simulink model "Drone_Simulation"  (R2020a)
settings: Solver=ode1  StartTime=0.0  StopTime=15  FixedStep=1e-3
undefined symbols (not defined in the file): AeEMSC, alpha1TDDBSC, B, bBNG, bEMSC, bEVCAP, BNG_Motor1, BNG_Motor2, BNG_Motor3, BNG_Motor4, BNG_Motor5, BNG_Motor6, bp, bq, br, bTDDBSC, bWDG, C_A, C_mot, C_th_esc, CAPEV_Motor1, CAPEV_Motor2, CAPEV_Motor3, CAPEV_Motor4, CAPEV_Motor5, CAPEV_Motor6, cdx, cdy, cdz, EaEMSC, EaEVCAP, EalphaTDDBSC, EaTDDBSC, EaWDG, FuselageContactForces, g, JrefEMSC, k_b, Kp, Kp2, Kq, Kq2, Kr, Kr2, kv, Kx, Ky, Kz, Kz2, LeftAftArm, LeftAftSkid, LeftArm, LeftFrontArm, LeftFrontSkid, LeftSideContactForces, LnomEMSC, LnomEVCAP, LnomTDDBSC, LnomWDG, Lower ... (+65)
libraries: sm_lib x90, nesl_utility x76, fl_lib x59, ee_lib x18, batteryecm_lib x2, dspinverses x1, dspmtrx3 x1
(part 1 of 5)
settings Model: Creator=G_MAMAN  LastModifiedBy=Asus
settings SolverCC: MaxConsecutiveZCs=100  ExtrapolationOrder=2  AlgebraicLoopSolver=LineSearch  SolverResetMethod=Robust
settings DataIOCC: LimitDataPoints=on  MaxDataPoints=10000  Refine=5
settings OptimizationCC: LifeSpan=inf
settings DebuggingCC: MaskedZcDiagnostic=none  IgnoredZcDiagnostic=none  AllowSymbolicDim=off  SFUnexpectedBacktrackingDiag=warning  SFNoUnconditionalDefaultTransitionDiag=warning  SFExecutionAtInitializationDiag=none  ArithmeticOperatorsInVariantConditions=warning
settings SFSimCC: SimUseLocalCustomCode=off  CustomCodeUndefinedFunction=UseInterfaceOnly
settings RTWCC: RTWUseLocalCustomCode=off
settings CodeAppCC: StateflowObjectComments=on
settings GRTTargetCC: TargetLangStandard=C89/C90 (ANSI)
settings ConfigComp: CovMetricSettings=dw  CovSaveCumulativeToWorkspaceVar=on  CovSaveSingleToWorkspaceVar=on  CovExternalEMLEnable=off  CovSFcnEnable=off
settings SimscapeCC: ExplicitSolverDiagnosticOptions=none  SimscapeLogType=all  SimscapeLogSimulationStatistics=on  SimscapeLogDataHistory=10000
settings DiagnosticsConfigSet: SimMechanicsRigidlyBoundBlock=none
settings ExplorerConfigSet: InternalSimMechanicsExplorerSettings="<ExplorerConfiguration><canonicalview>default</canonicalview><AnimationSetting><BasePlaybackSpeed>1.0</BasePlaybackSpeed><PlaybackSpeedFactor>1.0</PlaybackSpeedFactor></AnimationSetting><TilePanel><TileInfo><Tiles Columns=\"1\" Count=\"1\" Rows=\"1\"><Column Weight=\"1\"/><Row Weight=\"1\"/><Tile Height=\"1\" Width=\"1\" X=\"0\" Y=\"0\"/></Tiles></TileInfo><SceneInfo><SceneViewer><BGColor><R>0</R><G>0</G><B>0</B></BGColor><Camera><DoPerspective>off</DoPerspective><Position><X>7.1395388580893373</X><Y>-9.57545541238177833</Y><Z>5.80767107239631564</Z></Position><Center><X>-0.863567299281931766</X><Y>0.176174380151177173</Y><Z>1.92916926391305155</Z></Center><Up><X>-0.173509302469238902</X><Y>0.237715937307242831</Y><Z>0.955712119367949198</Z></Up><ViewLimDist>1</ViewLimDist><YLim>4.19925208742349287</YLim><XLim>9.96419089960335391</XLim></Camera></SceneViewer></SceneInfo></TilePanel><MechEditorPanel><Cameras/><GfxPanelCameraMap/><VideoCreator><PlaybackSpeedRatio>1.0</PlaybackSpeedRatio><FrameRate>30</FrameRate><VideoFormat>Motion JPEG AVI</VideoFormat><FrameSize>auto</FrameSize></VideoCreator></MechEditorPanel></ExplorerConfiguration>"

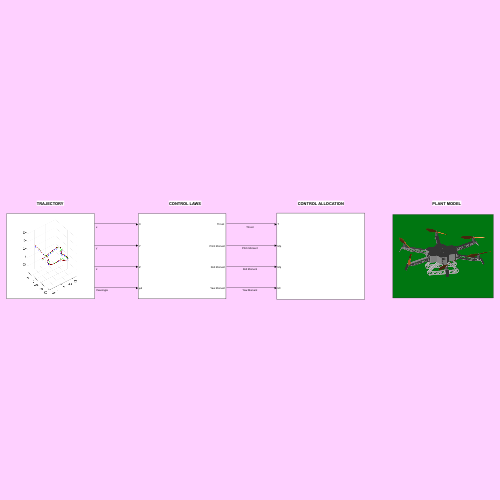
[thumbnail: Simulink's stored preview of the top-level diagram]
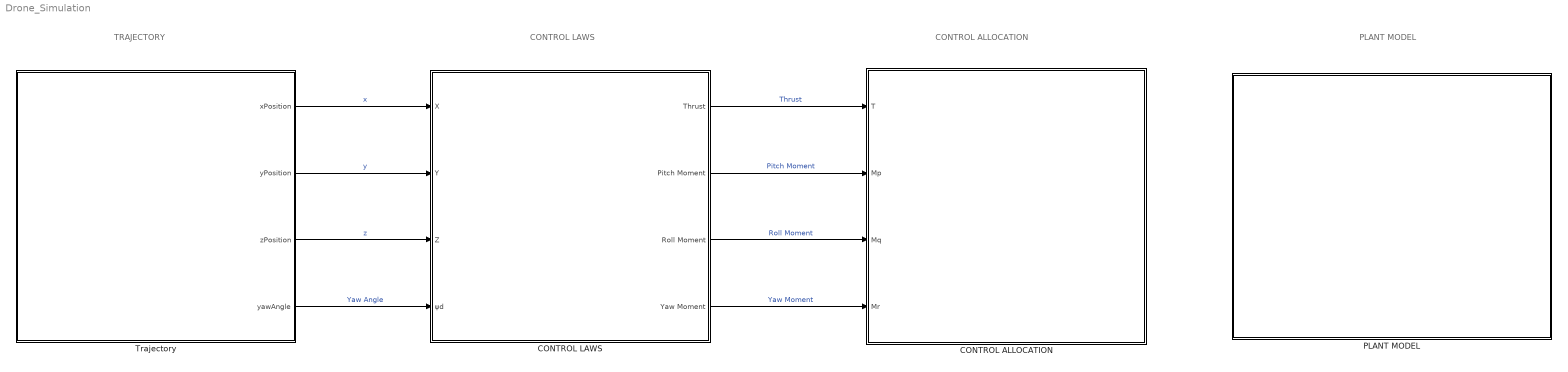
== system Drone_Simulation ==
  note: CONTROL LAWS
  note: CONTROL ALLOCATION
  note: PLANT MODEL
  note: TRAJECTORY
  CONTROL ALLOCATION : Subsystem
  CONTROL LAWS : Subsystem
  PLANT MODEL : Subsystem
      mask Display: image('$imagefile'); % Use "Edit Image" on toolstrip to change.
  Trajectory : Subsystem
      mask Display: image('$imagefile'); % Use "Edit Image" on toolstrip to change.
  wires:
  CONTROL LAWS/4(Yaw Moment) -> CONTROL ALLOCATION/4(Mr)  "Yaw Moment"
  CONTROL LAWS/2(Pitch Moment) -> CONTROL ALLOCATION/2(Mp)  "Pitch Moment"
  CONTROL LAWS/1("Thrust ") -> CONTROL ALLOCATION/1(T)  "Thrust"
  CONTROL LAWS/3(Roll Moment) -> CONTROL ALLOCATION/3(Mq)  "Roll Moment"
  Trajectory/1(xPosition) -> CONTROL LAWS/1(X)  "x"
  Trajectory/2(yPosition) -> CONTROL LAWS/2(Y)  "y"
  Trajectory/3(zPosition) -> CONTROL LAWS/3(Z)  "z"
  Trajectory/4(yawAngle) -> CONTROL LAWS/4(ψd)  "Yaw Angle"

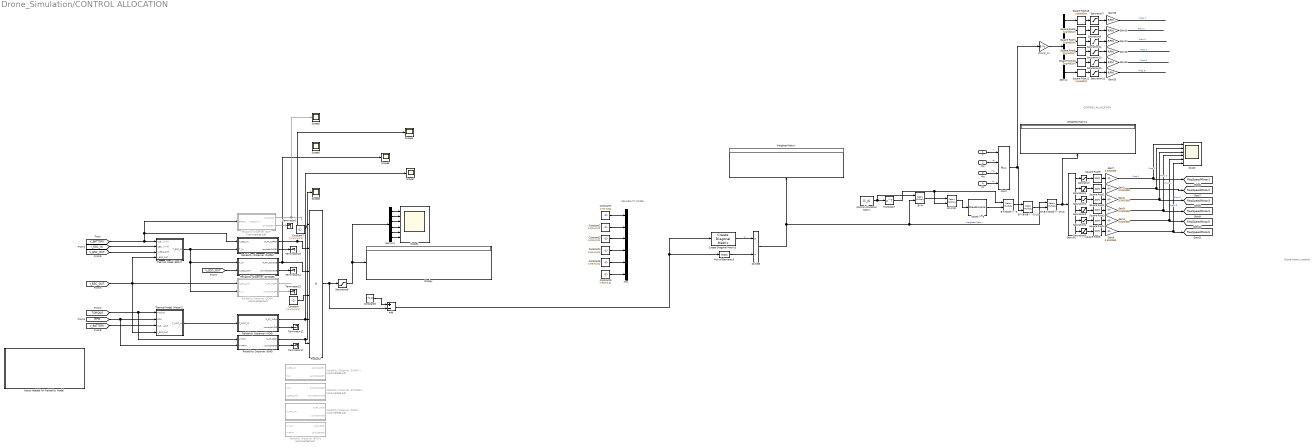
== system Drone_Simulation/CONTROL ALLOCATION ==
  note: Drone Motors Location
  note: RELIABILITY MODEL
  note: CONTROL ALLOCATION
  T : Inport
  Mp : Inport  Port=2
  Mq : Inport  Port=3
  Mr : Inport  Port=4
  (BWB')^-3 : dspinverses/Pseudoinverse  wanterr=off  SimulateUsing=Interpreted execution
  Add : Sum  Inputs=+-
  B'*(BWB')^-1*U3 : Product  Multiplication=Matrix(*)
  B'*(BWB')^-3 : Product  Multiplication=Matrix(*)
  B*W : Product  Multiplication=Matrix(*)
  B*W*B' : Product  Multiplication=Matrix(*)
  Constant : Constant  Value=[1,1,1,1,1,1]
  Constant1 : Constant  Value=1-R1+eps
  Constant2 : Constant  Value=1-R2+0.01
  Constant3 : Constant  Value=1-R3+0.01
  Constant4 : Constant  Value=1-R4+0.01
  Constant5 : Constant  Value=1-R5+0.01
  Constant6 : Constant  Value=1-R6+0.01
  Constant7 : Constant  Value=[1,1,1,1,1,1]
  Constant8 : Constant  Value=1+0.01
  Control Allocation Matrix : Constant  Value=[C_A]
  Create Diagonal Matrix3 : dspmtrx3/Create Diagonal Matrix
  Demux : Demux  Outputs=6
  Demux1 : Demux  Outputs=6
  Demux2 : Demux  Outputs=6
  Display : Display
  Divide3 : Product  Inputs=*/
  Gain{1..5,7} (6 alike) : Gain  Gain=9.5492968
  Gain{15..20} (6 alike) : Gain  Gain=RPM
  Inputs Needed For Reliability Model : Subsystem
  Max of Elements3 : MinMax  Function=max
  Mux : Mux  Inputs=6
  Mux2 : Mux
      settings: DisplayOption=signals
  Pinv(C_A) : Gain  Gain=B  Multiplication=Matrix(K*u)
  Product2 : Product  Inputs=6
  Reliability Observer (BAT) : Subsystem  Commented=on
  Reliability Observer (BNG) : Subsystem
  Reliability Observer (BNG)1 : Subsystem  Commented=on
  Reliability Observer (CAPEV) : Subsystem
  Reliability Observer (CAPEV)1 : Subsystem  Commented=on
  Reliability Observer (SCEM) : Subsystem  Commented=on
  Reliability Observer (SCTDDB) : Subsystem
  Reliability Observer (SCTDDB)1 : Subsystem  Commented=on
  Reliability Observer (WDG) : Subsystem
  Reliability Observer (WDG)1 : Subsystem  Commented=on
  Saturation{,1..5} (6 alike) : Saturate  UpperLimit=1096623  LowerLimit=0
  Saturation{7,9..13} (6 alike) : Saturate  UpperLimit=10000*(2*pi)/60  LowerLimit=0
  Saturation8 : Saturate  UpperLimit=1  LowerLimit=0.01
  Scope : Scope  NumInputPorts=6
  Scope1 : Scope  NumInputPorts=6
  Scope{3..8} (6 alike) : Scope
  Square Root{1..5,9} (6 alike) : Sqrt  SaturateOnIntegerOverflow=on
  Square Root{6..8,10..11,18} (6 alike) : Sqrt  Operator=signedSqrt  SaturateOnIntegerOverflow=on
  Terminator{1,12..15,17} (6 alike) : Terminator
  Thermal Model (ESC)2 : Subsystem
  Thermal Model (Motor)2 : Subsystem
  Transpose : Math  Operator=transpose  SaturateOnIntegerOverflow=on
  W*B'*(BWB')^-1*U3 : Product  Multiplication=Matrix(*)
  Weighted Matrix : Display
  Weighted Matrix1 : Display
  tag scope: ReqSpeedMotor1=global, ReqSpeedMotor2=global, ReqSpeedMotor3=global, ReqSpeedMotor4=global, ReqSpeedMotor5=global, ReqSpeedMotor6=global
  wires:
  B'*(BWB')^-1*U3/1 -> W*B'*(BWB')^-1*U3/2
  [RPM] -> Reliability Observer (BNG)/2(N (RPM)), Thermal Model (Motor)2/2(RPM)
  Thermal Model (Motor)2/1(T_MOT_IN) -> Reliability Observer (WDG)/1(T_MOT_IN)
  Demux2/6 -> Saturation5/1
  [V_BATTERY] -> Reliability Observer (CAPEV)/1(V_ESC_IN), Reliability Observer (BAT)/1(Battery Voltage (V)), Thermal Model (ESC)2/1(V_ESC_in (V))
  [I_ESC_IN] -> Thermal Model (ESC)2/2(I_ESC_in (A))
  [I_ESC_OUT] -> Reliability Observer (SCEM)/1(I_ESC_OUT), Thermal Model (ESC)2/4(I_ESC_OUT), Thermal Model (Motor)2/4(I_ESC_OUT)
  Square Root4/1 -> Gain4/1
  Demux2/2 -> Saturation1/1
  Mux2/1 -> Pinv(C_A)/1, B'*(BWB')^-1*U3/2
  [V_BATTERY] -> Thermal Model (Motor)2/3(V_ESC_OUT)
  Reliability Observer (SCEM)/2(LambdaSCEM) -> Terminator13/1
  Create Diagonal Matrix3/1 -> Divide3/1  "W"
  Square Root5/1 -> Gain5/1
  Transpose/1 -> B*W*B'/2, B'*(BWB')^-3/1
  B'*(BWB')^-3/1 -> B'*(BWB')^-1*U3/1
  Square Root3/1 -> Gain3/1
  [V_ESC_OUT] -> Thermal Model (ESC)2/3(V_ESC_OUT)
  Gain7/1 -> [ReqSpeedMotor1], Scope/1  "Prop 1"
  Reliability Observer (WDG)/2(LambdaWDG) -> Terminator12/1
  Demux2/4 -> Saturation3/1
  Reliability Observer (BNG)/2(LambdaBNG) -> Terminator17/1
  Control Allocation Matrix/1 -> B*W/1, Transpose/1
  Demux2/1 -> Saturation/1
  Reliability Observer (CAPEV)/2(LambdaCAPEV) -> Terminator15/1
  Gain3/1 -> [ReqSpeedMotor4], Scope/4  "Prop 4"
  Gain5/1 -> [ReqSpeedMotor6], Scope/6  "Prop 6"
  Gain4/1 -> [ReqSpeedMotor5], Scope/5  "Prop 5"
  [TORQUE] -> Reliability Observer (BNG)/1(M (Nm)), Thermal Model (Motor)2/1(Torque)
  Square Root1/1 -> Gain1/1
  Gain2/1 -> [ReqSpeedMotor3], Scope/3  "Prop 3"
  (BWB')^-3/1 -> B'*(BWB')^-3/2
  B*W/1 -> B*W*B'/1
  Square Root2/1 -> Gain2/1
  Gain1/1 -> [ReqSpeedMotor2], Scope/2  "Prop 2"
  Demux2/5 -> Saturation4/1
  Square Root9/1 -> Gain7/1
  Thermal Model (ESC)2/1(T_ESC_IN) -> Reliability Observer (CAPEV)/2(T_IN), Reliability Observer (SCTDDB)/1(T_IN), Reliability Observer (SCEM)/2(T_IN)
  Demux2/3 -> Saturation2/1
  Max of Elements3/1 -> Divide3/2
  Reliability Observer (SCTDDB)/2(LambdaSCTDDB) -> Terminator14/1
  Divide3/1 -> Weighted Matrix/1, B*W/2, W*B'*(BWB')^-1*U3/1  "Weighted Matrix"
  B*W*B'/1 -> (BWB')^-3/1
  Saturation/1 -> Square Root9/1
  Saturation1/1 -> Square Root1/1
  Saturation2/1 -> Square Root2/1
  Saturation3/1 -> Square Root3/1
  Saturation4/1 -> Square Root4/1
  Saturation5/1 -> Square Root5/1
  W*B'*(BWB')^-1*U3/1 -> Weighted Matrix1/1, Demux2/1
  T/1 -> Mux2/1  "T"
  Mp/1 -> Mux2/2  "Mp"
  Mq/1 -> Mux2/3  "Mq"
  Mr/1 -> Mux2/4  "Mr"
  [V_ESC_OUT] -> Reliability Observer (SCTDDB)/2(V_ESC_OUT)
  Reliability Observer (CAPEV)/1(R_RT_CAPEV) -> Scope4/1, Product2/2
  Reliability Observer (SCTDDB)/1(R_RT_SCTDDB) -> Product2/3, Scope6/1
  Reliability Observer (BNG)/1(R_RT_BNG) -> Scope8/1, Product2/6
  Reliability Observer (WDG)/1(R_RT_WDG) -> Scope7/1, Product2/5
  Reliability Observer (BAT)/2(LambdaBAT) -> Terminator1/1
  Reliability Observer (BAT)/1(R_RT_BAT) -> Scope3/1
  Constant/1 -> Product2/4
  Product2/1 -> Add/2, Saturation8/1
  Saturation11/1 -> Gain20/1
  Saturation10/1 -> Gain19/1
  Saturation9/1 -> Gain16/1
  Saturation13/1 -> Gain18/1
  Saturation12/1 -> Gain17/1
  Square Root6/1 -> Saturation9/1
  Square Root18/1 -> Saturation7/1
  Square Root8/1 -> Saturation13/1
  Square Root10/1 -> Saturation10/1
  Saturation7/1 -> Gain15/1
  Demux/4 -> Square Root8/1
  Demux/6 -> Square Root11/1
  Square Root11/1 -> Saturation11/1
  Demux/3 -> Square Root7/1
  Square Root7/1 -> Saturation12/1
  Demux/5 -> Square Root10/1
  Pinv(C_A)/1 -> Demux/1
  Demux/1 -> Square Root18/1
  Demux/2 -> Square Root6/1
  Gain15/1 -> ?  "Prop 1"
  Gain16/1 -> ?  "Prop 2"
  Gain17/1 -> ?  "Prop 3"
  Gain18/1 -> ?  "Prop 4"
  Gain19/1 -> ?  "Prop 5"
  Gain20/1 -> ?  "Prop 6"
  Constant4/1 -> Mux/4
  Constant2/1 -> Mux/2
  Constant1/1 -> Mux/1
  Constant3/1 -> Mux/3
  Constant6/1 -> Mux/6
  Constant5/1 -> Mux/5
  Saturation8/1 -> Demux1/1, Display/1
  Reliability Observer (SCEM)/1(R_RT_SCEM) -> ?
  Demux1/1 -> Scope1/1
  Demux1/2 -> Scope1/2
  Demux1/3 -> Scope1/3
  Demux1/4 -> Scope1/4
  Demux1/5 -> Scope1/5
  Demux1/6 -> Scope1/6
  Constant7/1 -> Product2/1
  Constant8/1 -> Add/1
  Add/1 -> Max of Elements3/1, Create Diagonal Matrix3/1

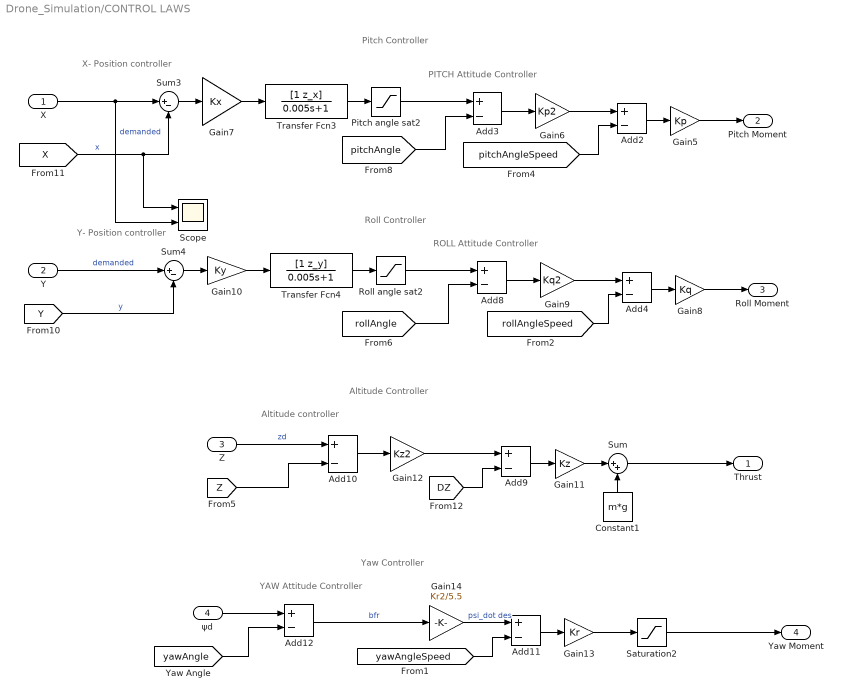
== system Drone_Simulation/CONTROL LAWS ==
  note: PITCH Attitude Controller
  note: X- Position controller
  note: YAW Attitude Controller
  note: Y- Position controller
  note: ROLL Attitude Controller
  note: Altitude controller
  note: Pitch Controller
  note: Roll Controller
  note: Altitude Controller
  note: Yaw Controller
  X : Inport
  Y : Inport  Port=2
  Z : Inport  Port=3
  ψd : Inport  Port=4
  Add{2..4,8..12} (8 alike) : Sum  Inputs=+-
  Constant1 : Constant  Value=m*g
  Gain10 : Gain  Gain=Ky
  Gain11 : Gain  Gain=Kz
  Gain12 : Gain  Gain=Kz2
  Gain13 : Gain  Gain=Kr
  Gain14 : Gain  Gain=Kr2/5.5
  Gain5 : Gain  Gain=Kp
  Gain6 : Gain  Gain=Kp2
  Gain7 : Gain  Gain=Kx
  Gain8 : Gain  Gain=Kq
  Gain9 : Gain  Gain=Kq2
  Pitch angle sat2 : Saturate  UpperLimit=pitch_angle_limit  LowerLimit=-pitch_angle_limit
  Roll angle sat2 : Saturate  UpperLimit=roll_angle_limit  LowerLimit=-roll_angle_limit
  Saturation2 : Saturate  UpperLimit=max_yaw_moment  LowerLimit=-max_yaw_moment
  Scope : Scope  NumInputPorts=2
  Sum : Sum  Inputs=|++
  Sum3 : Sum  Inputs=|+-
  Sum4 : Sum  Inputs=|+-
  Transfer Fcn3 : TransferFcn  Numerator=[1 z_x]  Denominator=[0.005 1]
  Transfer Fcn4 : TransferFcn  Numerator=[1 z_y]  Denominator=[0.005 1]
  "Thrust " : Outport
  Pitch Moment : Outport  Port=2
  Roll Moment : Outport  Port=3
  Yaw Moment : Outport  Port=4
  wires:
  Sum4/1 -> Gain10/1
  Add10/1 -> Gain12/1
  Add9/1 -> Gain11/1
  Add11/1 -> Gain13/1
  [DZ] -> Add9/2
  Transfer Fcn4/1 -> Roll angle sat2/1
  Add4/1 -> Gain8/1
  [Z] -> Add10/2
  Add12/1 -> Gain14/1  "bfr"
  Gain5/1 -> Pitch Moment/1
  Add2/1 -> Gain5/1
  Y/1 -> Sum4/1  "demanded"
  Gain10/1 -> Transfer Fcn4/1
  X/1 -> Scope/2, Sum3/1  "demanded"
  Roll angle sat2/1 -> Add8/1
  Sum/1 -> "Thrust "/1
  Constant1/1 -> Sum/2
  Gain9/1 -> Add4/1
  Transfer Fcn3/1 -> Pitch angle sat2/1
  Add8/1 -> Gain9/1
  Gain14/1 -> Add11/1  "psi_dot des"
  Gain6/1 -> Add2/1
  [yawAngle] -> Add12/2
  Add3/1 -> Gain6/1
  Z/1 -> Add10/1  "zd"
  Gain7/1 -> Transfer Fcn3/1
  Gain8/1 -> Roll Moment/1
  Sum3/1 -> Gain7/1
  Gain11/1 -> Sum/1
  Gain12/1 -> Add9/1
  ψd/1 -> Add12/1
  [Y] -> Sum4/2  "y"
  [rollAngle] -> Add8/2
  [rollAngleSpeed] -> Add4/2
  [X] -> Scope/1, Sum3/2  "x"
  [pitchAngle] -> Add3/2
  [pitchAngleSpeed] -> Add2/2
  Gain13/1 -> Saturation2/1
  Pitch angle sat2/1 -> Add3/1
  [yawAngleSpeed] -> Add11/2
  Saturation2/1 -> Yaw Moment/1

== system Drone_Simulation/PLANT MODEL ==
  BODY : Subsystem  mask{rgb=[0.753 0.753 0.753], op=1, rho=3400, H=0.051, D=0.235}
      mask prompts: rgb "Color of Fuselage [R G B]"; op "Opacity of Fuselage (0-1)"; rho "Density of Fuselage (kg/m^3)"; H "Height of Fuselage (m)"; D "Length of Fuselage (m)"
      mask Display: image('$imagefile'); % Use "Edit Image" on toolstrip to change.
  CONTACT FORCES : Subsystem  mask{st=4e5, b=4e4, trans=1e-4, mus=0.9, mud=0.8, vcr=1e-1}
      mask prompts: st "Stiffness (N/m)"; b "Damping (N/(m/s))"; trans "Transition Region Width (m)"; mus "Coefficient of Static Friction"; mud "Coefficient of Dynamic Friction"; vcr "Critical Velocity (m/s)"
      mask Display: image('$imagefile'); % Use "Edit Image" on toolstrip to change.
  Connection Label : ConnectionLabel  Label=LC
  Connection Label1 : ConnectionLabel  Label=RC
  Connection Label2 : ConnectionLabel  Label=SC
  Connection Label3 : ConnectionLabel  Label=PlantModel
  Connection Label4 : ConnectionLabel  Label=PlantModel
  Connection Label5 : ConnectionLabel  Label=LC
  Connection Label6 : ConnectionLabel  Label=RC
  Connection Label7 : ConnectionLabel  Label=SC
  DRAG FORCES : Subsystem
      mask Display: image('$imagefile'); % Use "Edit Image" on toolstrip to change.
  ELECTRIC SYSTEM : Subsystem  mask{Kv=1/930, R=0.136, Ic=0, J=0.000043, a=0.000110852, freq=10, Samp_time=1e-3}
      mask prompts: Kv "Voltage back emf Constant (v/rpm)"; R "Resistance"; Ic "No Load Current (A)"; J "Inertia (kg*m^2)"; a "Torque Coefficient (N/rpm)"; freq "PWM Frequency"; Samp_time "PWM Sample Time"
      mask DialogControl Motors Prompt: Motors
      mask DialogControl Propellers Prompt: Propellers
      mask DialogControl Container3 Prompt: Electronic Speed Controller
      mask Display: image('$imagefile'); % Use "Edit Image" on toolstrip to change.
  ENVIRONMENT : Subsystem  mask{E=20, P=0.1, Z=0.12}
      mask prompts: E "Size of Ground (m)"; P "Height of Ground (m)"; Z "Displacement of Ground (m)"
      mask Display: image('$imagefile'); % Use "Edit Image" on toolstrip to change.
  Fuselage Contact : ConnectionLabel  Label=FC
  Fuselage Contact1 : ConnectionLabel  Label=FC
  Mechanism Configuration : sm_lib/Utilities/Mechanism Configuration  UniformGravity=Constant  GravityVector=[0 0 -g]  GravityVectorUnits=m/s^2  LinearizationDelta=0.001  JointModeTransitionNonlinearIterations=2
  PROPELLER AND ARMS : Subsystem
      mask Display: image('$imagefile'); % Use "Edit Image" on toolstrip to change.
  Reference Frame : sm_lib/Frames and Transforms/Reference Frame
  SENSORS : Subsystem
      mask Display: image('$imagefile'); % Use "Edit Image" on toolstrip to change.
  Simscape Bus : SimscapeBus  HierarchyStrings=FuselageContactForces;LeftSideContactForces;RightSideContactForces;SkidsContactForces
  Solver Configuration : nesl_utility/Solver Configuration  PhysicalDomain=network_engine_domain  SubClassName=solver  LeftPortType=input  RightPortType=generic  Tones=[]  Harmonics=[]  SimulateNoise=off  Profile=off  UseLocalSampling=off  EnableSwitchedLinearOptims=on  FrequencyDomain=off  UseCCode=off  RelTol=0.001  AbsTol=0.001  MinStep=1e-09  ToWorkspace=off  RevertToSquareIcSolve=off  NumHomotopyIterations=100  PhasorMode=off  PhasorModeNumHarmonics=1  ConsistencySolver=NEWTON_FTOL  IndexReductionMethod=DerivativeReplacement  DoDC=off  ResidualTolerance=1e-09  ConsistencyTolSource=GLOBAL  ConsistencyAbsTol=0.001  ConsistencyRelTol=0.001  ConsistencyTolFactor=0.001  UseLocalSolver=off  LocalSolverChoice=NE_BACKWARD_EULER_ADVANCER  ResolveIndetEquations=on  FunctionEvalNumThread=1  LocalSolverSampleTime=0.001  DoFixedCost=off  MaxNonlinIter=3  MaxModeIter=2  ComputeImpulses=off  ImpulseIterations=2  LinearAlgebra=auto  LinearAlgebraNumThread=0  EquationFormulation=NE_TIME_EF  DelaysMemoryBudget=1024  AutomaticFiltering=on  FilteringTimeConstant=0.001  PartitionStorageMethod=AS_NEEDED  PartitionMemoryBudget=1024  PartitionMethod=ROBUST
  connections:
  Fuselage Contact/LConn1 -- BODY/LConn1
  BODY/RConn1 -- PROPELLER AND ARMS/RConn1 -- DRAG FORCES/RConn1 -- Solver Configuration/RConn1 -- Mechanism Configuration/RConn1 -- Connection Label4/LConn1 -- Reference Frame/RConn1
  Connection Label/LConn1 -- PROPELLER AND ARMS/RConn2
  Connection Label1/LConn1 -- PROPELLER AND ARMS/RConn3
  Connection Label3/LConn1 -- SENSORS/RConn1
  Fuselage Contact1/LConn1 -- Simscape Bus/LConn1
  Simscape Bus/LConn2 -- Connection Label5/LConn1
  Connection Label6/LConn1 -- Simscape Bus/LConn3
  Simscape Bus/LConn4 -- Connection Label7/LConn1
  Simscape Bus/RConn1 -- CONTACT FORCES/RConn2
  ENVIRONMENT/LConn1 -- CONTACT FORCES/RConn1
  ENVIRONMENT/RConn1 -- SENSORS/RConn2
  Connection Label2/LConn1 -- BODY/LConn2

== system Drone_Simulation/Trajectory ==
  Clock : Clock
  Constant : Constant  Value=timeConstant
  Constant1 : Constant  Value=missionPlanX
  Constant2 : Constant  Value=missionPlanY
  Constant4 : Constant  Value=missionPlanYaw
  Constant5 : Constant  Value=missionPlanZ
  Degrees to Rad : Gain  Gain=0.0174533
  Trajectory Control : MATLAB Function  TreatAsAtomicUnit=on
  xPosition : Outport
  yPosition : Outport  Port=2
  zPosition : Outport  Port=3
  yawAngle : Outport  Port=4
  wires:
  Trajectory Control/1(xPosition) -> xPosition/1
  Constant/1 -> Trajectory Control/5(timeConstant)
  Constant2/1 -> Trajectory Control/2(missionPlanY)
  Trajectory Control/3(zPosition) -> zPosition/1
  Trajectory Control/2(yPosition) -> yPosition/1
  Clock/1 -> Trajectory Control/6(simulationTime)
  Constant4/1 -> Degrees to Rad/1
  Degrees to Rad/1 -> Trajectory Control/4(missionPlanYaw)
  Trajectory Control/4(yaw) -> yawAngle/1
  Constant5/1 -> Trajectory Control/3(missionPlanZ)
  Constant1/1 -> Trajectory Control/1(missionPlanX)

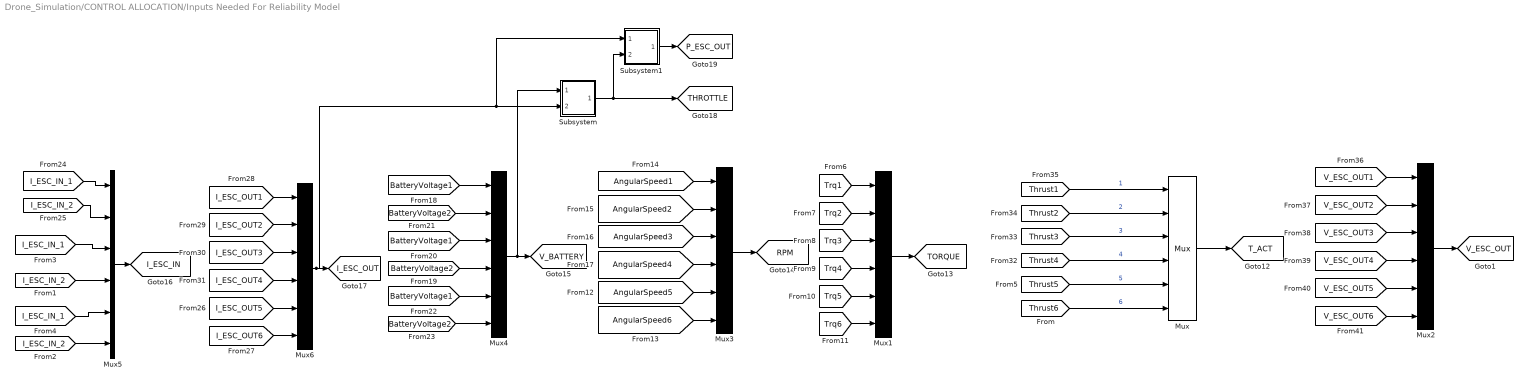
== system Drone_Simulation/CONTROL ALLOCATION/Inputs Needed For Reliability Model ==
  Mux{,1..6} (7 alike) : Mux  Inputs=6
  Subsystem : Subsystem
  Subsystem1 : Subsystem
  tag scope: I_ESC_IN=global, I_ESC_OUT=global, P_ESC_OUT=global, RPM=global, THROTTLE=global, TORQUE=global, T_ACT=global, V_BATTERY=global, V_ESC_OUT=global
  wires:
  [I_ESC_OUT4] -> Mux6/4
  [Trq2] -> Mux1/2
  Subsystem/1(Out1) -> Subsystem1/2(In2), [THROTTLE]
  [I_ESC_OUT5] -> Mux6/5
  [Trq5] -> Mux1/5
  [I_ESC_IN_1] -> Mux5/5
  [AngularSpeed4] -> Mux3/4
  [Trq1] -> Mux1/1
  [Thrust5] -> Mux/5  "5"
  [AngularSpeed1] -> Mux3/1
  [BatteryVoltage1] -> Mux4/1
  [I_ESC_OUT2] -> Mux6/2
  [I_ESC_OUT3] -> Mux6/3
  Mux6/1 -> Subsystem1/1(In1), Subsystem/2(In2), [I_ESC_OUT]
  [Thrust2] -> Mux/2  "2"
  [I_ESC_IN_1] -> Mux5/3
  Mux1/1 -> [TORQUE]
  [Thrust3] -> Mux/3  "3"
  [BatteryVoltage2] -> Mux4/2
  [Thrust6] -> Mux/6  "6"
  [AngularSpeed3] -> Mux3/3
  [AngularSpeed5] -> Mux3/5
  Mux5/1 -> [I_ESC_IN]
  [BatteryVoltage2] -> Mux4/6
  [I_ESC_IN_1] -> Mux5/1
  [I_ESC_OUT1] -> Mux6/1
  [Trq3] -> Mux1/3
  [Trq6] -> Mux1/6
  [BatteryVoltage2] -> Mux4/4
  Mux/1 -> [T_ACT]
  Mux3/1 -> [RPM]
  [I_ESC_IN_2] -> Mux5/6
  [Thrust4] -> Mux/4  "4"
  [Thrust1] -> Mux/1  "1"
  [I_ESC_OUT6] -> Mux6/6
  [AngularSpeed2] -> Mux3/2
  Subsystem1/1(Out1) -> [P_ESC_OUT]
  [Trq4] -> Mux1/4
  [I_ESC_IN_2] -> Mux5/2
  [I_ESC_IN_2] -> Mux5/4
  [AngularSpeed6] -> Mux3/6
  [BatteryVoltage1] -> Mux4/5
  [BatteryVoltage1] -> Mux4/3
  Mux4/1 -> Subsystem/1(In1), [V_BATTERY]
  [V_ESC_OUT4] -> Mux2/4
  [V_ESC_OUT6] -> Mux2/6
  Mux2/1 -> [V_ESC_OUT]
  [V_ESC_OUT3] -> Mux2/3
  [V_ESC_OUT2] -> Mux2/2
  [V_ESC_OUT5] -> Mux2/5
  [V_ESC_OUT1] -> Mux2/1

== system Drone_Simulation/CONTROL ALLOCATION/Reliability Observer (BAT) ==
  Battery Voltage (V) : Inport
  1-D Lookup Table : Lookup_n-D  NumberOfTableDimensions=1  BreakpointsForDimension1=[-4.99;-4.98;-4.97;-4.96;-4.95;-4.94;-4.93;-4.92;-4.91;-4.9;-4.89;-4.88;-4.87;-4.86;-4.85;-4.84;-4.83;-4.82;-4.81;-4.8;-4.79;-4.78;-4.77;-4.76;-4.75;-4.74;-4.73;-4.72;-4.71;-4.7;-4.69;-4.68;-4.67;-4.66;-4.65;-4.64;-4.63;-4.62;-4.61;-4.6;-4.59;-4.58;-4.57;-4.56;-4.55;-4.54;-4.53;-4.52;-4.51;-4.5;-4.49;-4.48;-4.47;-4.46;-4.45;-4.44;-4.43;-4.42;-4.41;-4.4;-4.39;-4.38;-4.37;-4.36;-4.35;-4.34;-4.33;-4.32;-4.31;-4.3;-4.29;-4.28;-4.27;-4.26;-4.25;-4.24;-4.23;-4.22;-4.21;-4.2;-4.19;-4.18;-4.17;-4.16;-4.15;-4.14;-4.13;-4.12;-4.11;-4.1;-4.09;-4.08;-4.07;-4.06;-4.05;-4.04;-4.03;-4.02;-4.01;-4;-3.99;-3.98;-3.97;-3.96;-3.95;-3.94;-3.93;-3.92;-3.91;-3.9;-3.89;-3.88;-3.87;-3.86;-3.85;-3.84;-3.83;-3.82;-3.81;-3.8;-3.79;-3.78;-3.77;-3.76;-3.75;-3.74;-3.73;-3.72;-3.71;-3.7;-3.69;-3.68;-3.67;-3.66;-3.65;-3.64;-3.63;-3.62;-3.61;-3.6;-3.59;-3.58;-3.57;-3.56;-3.55;-3.54;-3.53;-3.52;-3.51;-3.5;-3.49;-3.48;-3.47;-3.46;-3.45;-3.44;-3.43;-3.42;-3.41;-3.4;-3.39;-3.38;-3.37;-3.36;-3.35;-3.34;-3.33;-3.32;-3.31;-3.3;-3.29;-3.28;-3.27;-3.26;-3.25;-3.24;-3.23;-3.22;-3.21;-3.2;-3.19;-3.18;-3.17;-3.16;-3.15;-3.14;-3.13;-3.12;-3.11;-3.1;-3.09;-3.08;-3.07;-3.06;-3.05;-3.04;-3.03;-3.02;-3.01;-3;-2.99;-2.98;-2.97;-2.96;-2.95;-2.94;-2.93;-2.92;-2.91;-2.9;-2.89;-2.88;-2.87;-2.86;-2.85;-2.84;-2.83;-2.82;-2.81;-2.8;-2.79;-2.78;-2.77;-2.76;-2.75;-2.74;-2.73;-2.72;-2.71;-2.7;-2.69;-2.68;-2.67;-2.66;-2.65;-2.64;-2.63;-2.62;-2.61;-2.6;-2.59;-2.58;-2.57;-2.56;-2.55;-2.54;-2.53;-2.52;-2.51;-2.5;-2.49;-2.48;-2.47;-2.46;-2.45;-2.44;-2.43;-2.42;-2.41;-2.4;-2.39;-2.38;-2.37;-2.36;-2.35;-2.34;-2.33;-2.32;-2.31;-2.3;-2.29;-2.28;-2.27;-2.26;-2.25;-2.24;-2.23;-2.22;-2.21;-2.2;-2.19;-2.18;-2.17;-2.16;-2.15;-2.14;-2.13;-2.12;-2.11;-2.1;-2.09;-2.08;-2.07;-2.06;-2.05;-2.04;-2.03;-2.02;-2.01;-2;-1.99;-1.98;-1.97;-1.96;-1.95;-1.94;-1.93;-1.92;-1.91;-1.9;-1.89;-1.88;-1.87;-1.86;-1.85;-1.84;-1.83;-1.82;-1.81;-1.8;-1.79;-1.78;-1.77;-1.76;-1.75;-1.74;-1.73;-1.72;-1.71;-1.7;-1.69;-1.68;-1.67;-1.66;-1.65;-1.64;-1.63;-1.62;-1.61;-1.6;-1.59;-1.58;-1.57;-1.56;-1.55;-1.54;-1.53;-1.52;-1.51;-1.5;-1.49;-1.48;-1.47;-1.46;-1.45;-1.44;-1.43;-1.42;-1.41;-1.4;-1.39;-1.38;-1.37;-1.36;-1.35;-1.34;-1.33;-1.32;-1.31;-1.3;-1.29;-1.28;-1.27;-1.26;-1.25;-1.24;-1.23;-1.22;-1.21;-1.2;-1.19;-1.18;-1.17;-1.16;-1.15;-1.14;-1.13;-1.12;-1.11;-1.1;-1.09;-1.08;-1.07;-1.06;-1.05;-1.04;-1.03;-1.02;-1.01;-1;-0.99;-0.98;-0.97;-0.96;-0.95;-0.94;-0.93;-0.92;-0.91;-0.9;-0.89;-0.88;-0.87;-0.86;-0.85;-0.84;-0.83;-0.82;-0.81;-0.8;-0.79;-0.78;-0.77;-0.76;-0.75;-0.74;-0.73;-0.72;-0.71;-0.7;-0.69;-0.68;-0.67;-0.66;-0.65;-0.64;-0.63;-0.62;-0.61;-0.6;-0.59;-0.58;-0.57;-0.56;-0.55;-0.54;-0.53;-0.52;-0.51;-0.5;-0.49;-0.48;-0.47;-0.46;-0.45;-0.44;-0.43;-0.42;-0.41;-0.4;-0.39;-0.38;-0.37;-0.36;-0.35;-0.34;-0.33;-0.32;-0.31;-0.3;-0.29;-0.28;-0.27;-0.26;-0.25;-0.24;-0.23;-0.22;-0.21;-0.2;-0.19;-0.18;-0.17;-0.16;-0.15;-0.14;-0.13;-0.12;-0.11;-0.1;-0.09;-0.08;-0.07;-0.06;-0.05;-0.04;-0.03;-0.02;-0.01;0]  Table=[3.019e-07;3.1792e-07;3.3476e-07;3.5247e-07;3.7107e-07;3.9061e-07;4.1115e-07;4.3272e-07;4.5538e-07;4.7918e-07;5.0418e-07;5.3043e-07;5.5799e-07;5.8693e-07;6.1731e-07;6.492e-07;6.8267e-07;7.1779e-07;7.5465e-07;7.9333e-07;8.3391e-07;8.7648e-07;9.2113e-07;9.6796e-07;1.0171e-06;1.0686e-06;1.1226e-06;1.1792e-06;1.2386e-06;1.3008e-06;1.366e-06;1.4344e-06;1.506e-06;1.581e-06;1.6597e-06;1.742e-06;1.8283e-06;1.9187e-06;2.0133e-06;2.1125e-06;2.2162e-06;2.3249e-06;2.4386e-06;2.5577e-06;2.6823e-06;2.8127e-06;2.9492e-06;3.092e-06;3.2414e-06;3.3977e-06;3.5612e-06;3.7322e-06;3.911e-06;4.098e-06;4.2935e-06;4.4979e-06;4.7117e-06;4.935e-06;5.1685e-06;5.4125e-06;5.6675e-06;5.934e-06;6.2123e-06;6.5031e-06;6.8069e-06;7.1241e-06;7.4555e-06;7.8015e-06;8.1627e-06;8.5399e-06;8.9337e-06;9.3447e-06;9.7736e-06;1.0221e-05;1.0689e-05;1.1176e-05;1.1685e-05;1.2215e-05;1.2769e-05;1.3346e-05;1.3948e-05;1.4575e-05;1.523e-05;1.5912e-05;1.6624e-05;1.7365e-05;1.8138e-05;1.8944e-05;1.9783e-05;2.0658e-05;2.1569e-05;2.2518e-05;2.3507e-05;2.4536e-05;2.5609e-05;2.6726e-05;2.7888e-05;2.9099e-05;3.0359e-05;3.1671e-05;3.3037e-05;3.4458e-05;3.5936e-05;3.7475e-05;3.9076e-05;4.0741e-05;4.2473e-05;4.4274e-05;4.6148e-05;4.8096e-05;5.0122e-05;5.2228e-05;5.4418e-05;5.6694e-05;5.9059e-05;6.1517e-05;6.4072e-05;6.6726e-05;6.9483e-05;7.2348e-05;7.5324e-05;7.8414e-05;8.1624e-05;8.4957e-05;8.8417e-05;9.201e-05;9.574e-05;9.9611e-05;0.00010363;0.0001078;0.00011213;0.00011662;0.00012128;0.00012611;0.00013112;0.00013632;0.00014171;0.0001473;0.0001531;0.00015911;0.00016534;0.0001718;0.00017849;0.00018543;0.00019262;0.00020006;0.00020778;0.00021577;0.00022405;0.00023263;0.00024151;0.00025071;0.00026023;0.00027009;0.00028029;0.00029086;0.00030179;0.00031311;0.00032481;0.00033693;0.00034946;0.00036243;0.00037584;0.00038971;0.00040406;0.00041889;0.00043423;0.00045009;0.00046648;0.00048342;0.00050094;0.00051904;0.00053774;0.00055706;0.00057703;0.00059765;0.00061895;0.00064095;0.00066367;0.00068714;0.00071136;0.00073638;0.00076219;0.00078885;0.00081635;0.00084474;0.00087403;0.00090426;0.00093544;0.0009676;0.00100078;0.001035;0.00107029;0.00110668;0.00114421;0.00118289;0.00122277;0.00126387;0.00130624;0.0013499;0.00139489;0.00144124;0.001489;0.0015382;0.00158887;0.00164106;0.00169481;0.00175016;0.00180714;0.00186581;0.00192621;0.00198838;0.00205236;0.00211821;0.00218596;0.00225568;0.0023274;0.00240118;0.00247707;0.00255513;0.0026354;0.00271794;0.00280281;0.00289007;0.00297976;0.00307196;0.00316672;0.0032641;0.00336416;0.00346697;0.0035726;0.00368111;0.00379256;0.00390703;0.00402459;0.0041453;0.00426924;0.00439649;0.00452711;0.00466119;0.0047988;0.00494002;0.00508493;0.00523361;0.00538615;0.00554262;0.00570313;0.00586774;0.00603656;0.00620967;0.00638715;0.00656912;0.00675565;0.00694685;0.00714281;0.00734363;0.00754941;0.00776025;0.00797626;0.00819754;0.00842419;0.00865632;0.00889404;0.00913747;0.00938671;0.00964187;0.00990308;0.01017044;0.01044408;0.01072411;0.01101066;0.01130384;0.01160379;0.01191063;0.01222447;0.01254546;0.01287372;0.01320938;0.01355258;0.01390345;0.01426212;0.01462873;0.01500342;0.01538633;0.01577761;0.01617738;0.01658581;0.01700302;0.01742918;0.01786442;0.0183089;0.01876277;0.01922617;0.01969927;0.02018222;0.02067516;0.02117827;0.02169169;0.02221559;0.02275013;0.02329547;0.02385176;0.02441919;0.0249979;0.02558806;0.02618984;0.02680342;0.02742895;0.02806661;0.02871656;0.02937898;0.03005404;0.03074191;0.03144276;0.03215677;0.03288412;0.03362497;0.0343795;0.03514789;0.03593032;0.03672696;0.03753798;0.03836357;0.0392039;0.04005916;0.04092951;0.04181514;0.04271622;0.04363294;0.04456546;0.04551398;0.04647866;0.04745968;0.04845723;0.04947147;0.05050258;0.05155075;0.05261614;0.05369893;0.05479929;0.0559174;0.05705343;0.05820756;0.05937994;0.06057076;0.06178018;0.06300836;0.06425549;0.06552171;0.0668072;0.06811212;0.06943662;0.07078088;0.07214504;0.07352926;0.0749337;0.07635851;0.07780384;0.07926984;0.08075666;0.08226444;0.08379332;0.08534345;0.08691496;0.08850799;0.09012267;0.09175914 ...(+1437 chars)]  InternalRulePriority=Speed  RndMeth=Simplest  InputSameDT=on
  Add : Sum
  Add1 : Sum  Inputs=+-
  Add2 : Sum  Inputs=+-
  Constant : Constant
  Divide : Product  Inputs=*/
  Gain : Gain  Gain=1/4
  Math Function : Math  Operator=pow  SaturateOnIntegerOverflow=on
  Math Function1 : Math  Operator=square  SaturateOnIntegerOverflow=on
  Math Function2 : Math  Operator=square  SaturateOnIntegerOverflow=on
  Mean_20%_SOC : Constant  Value=3.3488
  STD_Dev_20%_SOC : Constant  Value=0.0279
  STD_Dev_Measured_Voltage : Constant  Value=0.0333
  sqrt : Constant  Value=0.5
  R_RT_BAT : Outport
  LambdaBAT : Outport  Port=2
  wires:
  sqrt/1 -> Math Function/2
  STD_Dev_20%_SOC/1 -> Math Function2/1
  Add/1 -> Math Function/1
  STD_Dev_Measured_Voltage/1 -> Math Function1/1
  Math Function1/1 -> Add/2
  Math Function2/1 -> Add/1
  Math Function/1 -> Divide/2
  Battery Voltage (V)/1 -> Gain/1
  Mean_20%_SOC/1 -> Add1/1
  Constant/1 -> Add2/1
  Add2/1 -> R_RT_BAT/1
  Divide/1 -> 1-D Lookup Table/1
  1-D Lookup Table/1 -> Add2/2, LambdaBAT/1
  Gain/1 -> Add1/2
  Add1/1 -> Divide/1

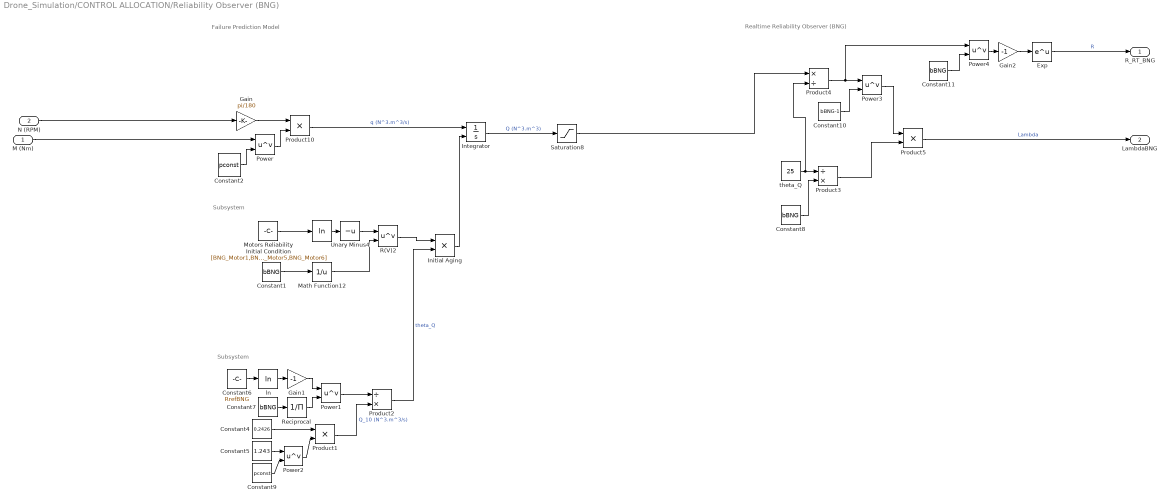
== system Drone_Simulation/CONTROL ALLOCATION/Reliability Observer (BNG) ==
  note: Subsystem
  note: Realtime Reliability Observer (BNG)
  note: Failure Prediction Model
  note: Subsystem
  M (Nm) : Inport
  N (RPM) : Inport  Port=2
  " " : Math  Operator=log  SaturateOnIntegerOverflow=on
  Constant{1,7..8,11} (4 alike) : Constant  Value=bBNG
  Constant10 : Constant  Value=bBNG-1
  Constant2 : Constant  Value=pconst
  Constant4 : Constant  Value=0.2426
  Constant5 : Constant  Value=1.243
  Constant6 : Constant  Value=RrefBNG
  Constant9 : Constant  Value=pconst
  Exp : Math  SaturateOnIntegerOverflow=on
  Gain : Gain  Gain=pi/180
  Gain1 : Gain  Gain=-1
  Gain2 : Gain  Gain=-1
  Initial Aging : Product
  Integrator : Integrator  InitialConditionSource=external  InitialCondition=[0;0;0;0;0;0]
  Math Function12 : Math  Operator=reciprocal  SaturateOnIntegerOverflow=on
  Motors Reliability Initial Condition : Constant  Value=[BNG_Motor1,BNG_Motor2,BNG_Motor3,BNG_Motor4,BNG_Motor5,BNG_Motor6]
  Power{,1..4} (5 alike) : Math  Operator=pow  SaturateOnIntegerOverflow=on
  Product1 : Product
  Product10 : Product
  Product2 : Product  Inputs=/*
  Product3 : Product  Inputs=/*
  Product4 : Product  Inputs=*/
  Product5 : Product
  R(V)2 : Math  Operator=pow  SaturateOnIntegerOverflow=on
  Reciprocal : Product  Inputs=/
  Saturation8 : Saturate  UpperLimit=1000000  LowerLimit=0
  Unary Minus4 : UnaryMinus
  ln : Math  Operator=log  SaturateOnIntegerOverflow=on
  theta_Q : Constant  Value=25
  R_RT_BNG : Outport
  LambdaBNG : Outport  Port=2
  wires:
  Gain/1 -> Product10/1
  N (RPM)/1 -> Gain/1
  Product10/1 -> Integrator/1  "q (N^3.m^3/s)"
  M (Nm)/1 -> Power/1
  Power/1 -> Product10/2
  Constant2/1 -> Power/2
  Exp/1 -> R_RT_BNG/1  "R"
  Constant11/1 -> Power4/2
  Product5/1 -> LambdaBNG/1  "Lambda"
  Gain2/1 -> Exp/1
  Constant8/1 -> Product3/2
  Product3/1 -> Product5/2
  Power4/1 -> Gain2/1
  Constant10/1 -> Power3/2
  theta_Q/1 -> Product4/2, Product3/1
  Product4/1 -> Power4/1, Power3/1
  Integrator/1 -> Saturation8/1  "Q (N^3.m^3)"
  Power3/1 -> Product5/1
  Constant9/1 -> Power2/2
  Constant5/1 -> Power2/1
  ln/1 -> Gain1/1
  Gain1/1 -> Power1/1
  Constant4/1 -> Product1/1
  Constant7/1 -> Reciprocal/1
  Product2/1 -> Initial Aging/2  "theta_Q"
  Power1/1 -> Product2/1
  Power2/1 -> Product1/2
  Reciprocal/1 -> Power1/2
  Product1/1 -> Product2/2  "Q_10 (N^3.m^3/s)"
  Constant6/1 -> ln/1
  Math Function12/1 -> R(V)2/2
  R(V)2/1 -> Initial Aging/1
  Constant1/1 -> Math Function12/1
  " "/1 -> Unary Minus4/1
  Unary Minus4/1 -> R(V)2/1
  Motors Reliability Initial Condition/1 -> " "/1
  Initial Aging/1 -> Integrator/2
  Saturation8/1 -> Product4/1

== system Drone_Simulation/CONTROL ALLOCATION/Reliability Observer (BNG)1 ==
  M (Nm) : Inport
  N (RPM) : Inport  Port=2
  Failure Prediction Model : Subsystem
  Realtime Reliability Observer (BNG) : Subsystem
  R_RT_BNG : Outport
  LambdaBNG : Outport  Port=2
  wires:
  Realtime Reliability Observer (BNG)/1(Lambda) -> LambdaBNG/1
  M (Nm)/1 -> Failure Prediction Model/2(M (Nm))
  Realtime Reliability Observer (BNG)/2(R) -> R_RT_BNG/1
  N (RPM)/1 -> Failure Prediction Model/1(N (RPM))
  Failure Prediction Model/1(q (N^3.m^3/s)) -> Realtime Reliability Observer (BNG)/1(q (N^3.m^3/s))

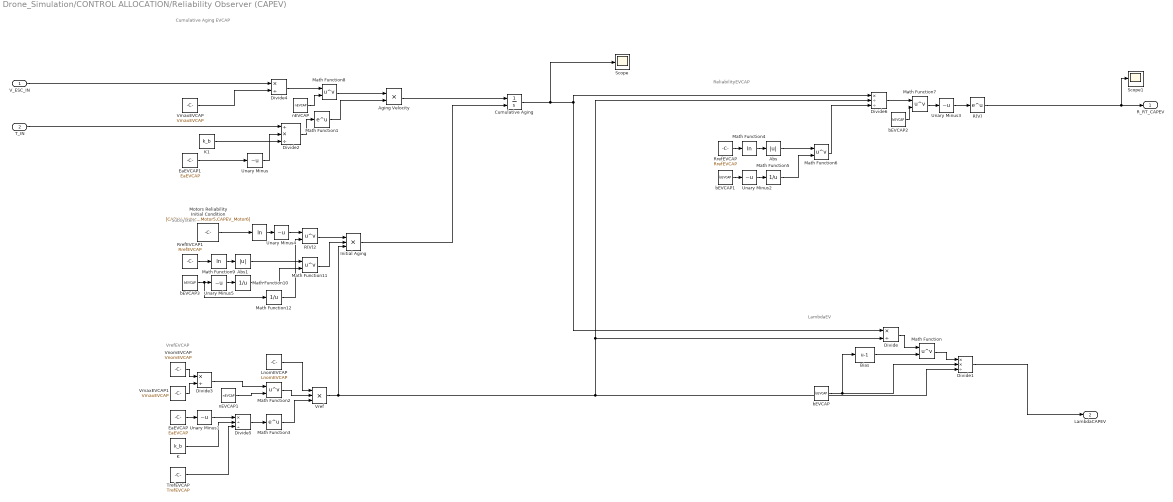
== system Drone_Simulation/CONTROL ALLOCATION/Reliability Observer (CAPEV) ==
  note: Subsystem
  note: Cumulative Aging EVCAP
  note: VrefEVCAP
  note: ReliabilityEVCAP
  note: LambdaEV
  V_ESC_IN : Inport
  T_IN : Inport  Port=2
  " " : Math  Operator=log  SaturateOnIntegerOverflow=on
  Abs : Abs
  Abs1 : Abs
  Aging Velocity : Product
  Bias : Bias  Bias=-1
  Cumulative Aging : Integrator  InitialConditionSource=external
  Divide : Product  Inputs=*/
  Divide1 : Product  Inputs=**/
  Divide2 : Product  Inputs=/*/
  Divide3 : Product  Inputs=*/
  Divide4 : Product  Inputs=*/
  Divide5 : Product  Inputs=*//
  Divide6 : Product  Inputs=*//
  EaEVCAP : Constant  Value=EaEVCAP
  EaEVCAP1 : Constant  Value=EaEVCAP
  Initial Aging : Product  Inputs=3
  K : Constant  Value=k_b
  K1 : Constant  Value=k_b
  LnomEVCAP : Constant  Value=LnomEVCAP
  Math Function{,2,6..8,11} (6 alike) : Math  Operator=pow  SaturateOnIntegerOverflow=on
  Math Function1 : Math  SaturateOnIntegerOverflow=on
  Math Function10 : Math  Operator=reciprocal  SaturateOnIntegerOverflow=on
  Math Function12 : Math  Operator=reciprocal  SaturateOnIntegerOverflow=on
  Math Function3 : Math  SaturateOnIntegerOverflow=on
  Math Function4 : Math  Operator=log  SaturateOnIntegerOverflow=on
  Math Function5 : Math  Operator=reciprocal  SaturateOnIntegerOverflow=on
  Math Function9 : Math  Operator=log  SaturateOnIntegerOverflow=on
  Motors Reliability Initial Condition : Constant  Value=[CAPEV_Motor1,CAPEV_Motor2,CAPEV_Motor3,CAPEV_Motor4,CAPEV_Motor5,CAPEV_Motor6]
  R(V) : Math  SaturateOnIntegerOverflow=on
  R(V)2 : Math  Operator=pow  SaturateOnIntegerOverflow=on
  RrefEVCAP : Constant  Value=RrefEVCAP
  RrefEVCAP1 : Constant  Value=RrefEVCAP
  Scope : Scope
  Scope1 : Scope
  TrefEVCAP : Constant  Value=TrefEVCAP
  Unary Minus{,1..5} (6 alike) : UnaryMinus
  VmaxEVCAP : Constant  Value=VmaxEVCAP
  VmaxEVCAP1 : Constant  Value=VmaxEVCAP
  VnomEVCAP : Constant  Value=VnomEVCAP
  Vref : Product  Inputs=3
  bEVCAP{,1..3} (4 alike) : Constant  Value=bEVCAP
  nEVCAP : Constant  Value=nEVCAP
  nEVCAP1 : Constant  Value=nEVCAP
  R_RT_CAPEV : Outport
  LambdaCAPEV : Outport  Port=2
  wires:
  Divide2/1 -> Math Function1/1
  Math Function/1 -> Divide1/1
  Bias/1 -> Math Function/2
  bEVCAP2/1 -> Math Function7/2
  Abs/1 -> Math Function6/1
  VmaxEVCAP/1 -> Divide4/2
  LnomEVCAP/1 -> Vref/1
  Math Function5/1 -> Math Function6/2
  nEVCAP1/1 -> Math Function2/2
  Divide4/1 -> Math Function8/1
  Math Function7/1 -> Unary Minus3/1
  bEVCAP1/1 -> Unary Minus2/1
  Math Function4/1 -> Abs/1
  Unary Minus3/1 -> R(V)/1
  V_ESC_IN/1 -> Divide4/1
  Divide6/1 -> Math Function7/1
  K1/1 -> Divide2/3
  Math Function6/1 -> Divide6/3
  TrefEVCAP/1 -> Divide5/3
  nEVCAP/1 -> Math Function8/2
  Aging Velocity/1 -> Cumulative Aging/1
  Unary Minus2/1 -> Math Function5/1
  VmaxEVCAP1/1 -> Divide3/2
  K/1 -> Divide5/2
  Unary Minus1/1 -> Divide5/1
  Math Function3/1 -> Vref/3
  Unary Minus/1 -> Divide2/2
  EaEVCAP1/1 -> Unary Minus/1
  Divide5/1 -> Math Function3/1
  VnomEVCAP/1 -> Divide3/1
  Divide3/1 -> Math Function2/1
  Math Function1/1 -> Aging Velocity/2
  Divide1/1 -> LambdaCAPEV/1
  Divide/1 -> Math Function/1
  Math Function2/1 -> Vref/2
  T_IN/1 -> Divide2/1
  Math Function8/1 -> Aging Velocity/1
  Cumulative Aging/1 -> Scope/1, Divide6/1, Divide/1
  EaEVCAP/1 -> Unary Minus1/1
  bEVCAP/1 -> Divide1/2, Bias/1
  RrefEVCAP/1 -> Math Function4/1
  Initial Aging/1 -> Cumulative Aging/2
  Math Function12/1 -> R(V)2/2
  R(V)2/1 -> Initial Aging/1
  Math Function10/1 -> Math Function11/2
  Vref/1 -> Divide/2, Divide6/2, Divide1/3, Initial Aging/3
  Unary Minus5/1 -> Math Function10/1
  Math Function9/1 -> Abs1/1
  " "/1 -> Unary Minus4/1
  RrefEVCAP1/1 -> Math Function9/1
  Unary Minus4/1 -> R(V)2/1
  Math Function11/1 -> Initial Aging/2
  Abs1/1 -> Math Function11/1
  bEVCAP3/1 -> Math Function12/1, Unary Minus5/1
  Motors Reliability Initial Condition/1 -> " "/1
  R(V)/1 -> Scope1/1, R_RT_CAPEV/1

== system Drone_Simulation/CONTROL ALLOCATION/Reliability Observer (CAPEV)1 ==
  V_ESC_IN : Inport
  T_IN : Inport  Port=2
  Cumulative Aging EVCAP : Subsystem
  LambdaEV : Subsystem
  ReliabilityEVCAP : Subsystem
  VrefEVCAP : Subsystem
  R_RT_CAPEV : Outport
  LambdaCAPEV : Outport  Port=2
  wires:
  ReliabilityEVCAP/1(Out1) -> R_RT_CAPEV/1
  T_IN/1 -> Cumulative Aging EVCAP/2(In3)
  V_ESC_IN/1 -> Cumulative Aging EVCAP/1(In1)
  Cumulative Aging EVCAP/1(Out1) -> LambdaEV/1(In1), ReliabilityEVCAP/1(In1)
  VrefEVCAP/1(Out1) -> LambdaEV/2(In2), ReliabilityEVCAP/2(In2), LambdaEV/3(In3)
  LambdaEV/1(Out1) -> LambdaCAPEV/1

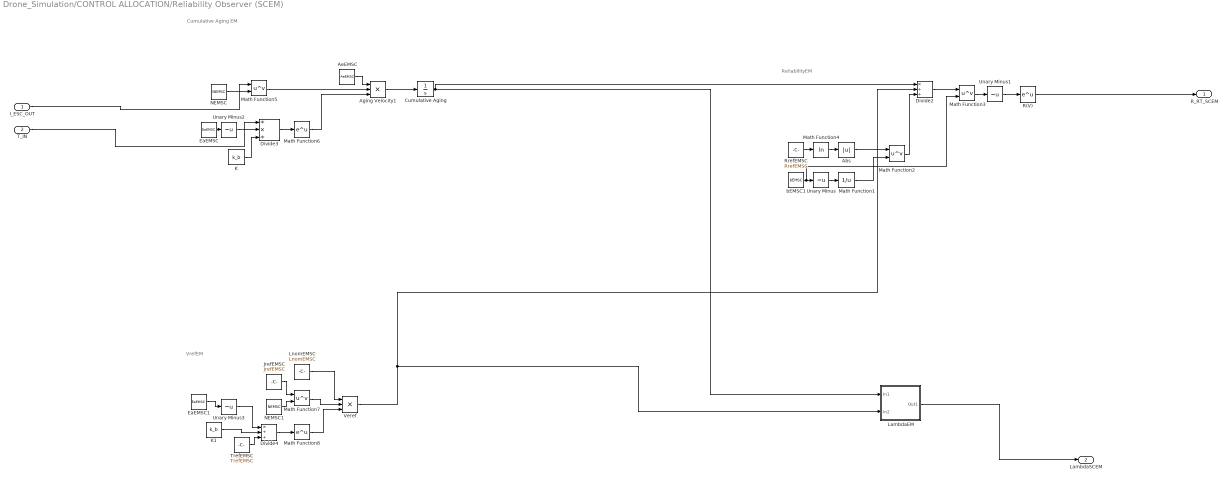
== system Drone_Simulation/CONTROL ALLOCATION/Reliability Observer (SCEM) ==
  note: ReliabilityEM
  note: VrefEM
  note: Cumulative Aging EM
  I_ESC_OUT : Inport
  T_IN : Inport  Port=2
  Abs : Abs
  AeEMSC : Constant  Value=AeEMSC
  Aging Velocity1 : Product  Inputs=3
  Cumulative Aging : Integrator
  Divide2 : Product  Inputs=*//
  Divide3 : Product  Inputs=/*/
  Divide4 : Product  Inputs=*//
  EaEMSC : Constant  Value=EaEMSC
  EaEMSC1 : Constant  Value=EaEMSC
  JrefEMSC : Constant  Value=JrefEMSC
  K : Constant  Value=k_b
  K1 : Constant  Value=k_b
  LambdaEM : Subsystem
  LnomEMSC : Constant  Value=LnomEMSC
  Math Function1 : Math  Operator=reciprocal  SaturateOnIntegerOverflow=on
  Math Function{2..3,5,7} (4 alike) : Math  Operator=pow  SaturateOnIntegerOverflow=on
  Math Function4 : Math  Operator=log  SaturateOnIntegerOverflow=on
  Math Function6 : Math  SaturateOnIntegerOverflow=on
  Math Function8 : Math  SaturateOnIntegerOverflow=on
  NEMSC : Constant  Value=NEMSC
  NEMSC1 : Constant  Value=NEMSC
  R(V) : Math  SaturateOnIntegerOverflow=on
  RrefEMSC : Constant  Value=RrefEMSC
  TrefEMSC : Constant  Value=TrefEMSC
  Unary Minus{,1..3} (4 alike) : UnaryMinus
  Veref : Product  Inputs=3
  bEMSC1 : Constant  Value=bEMSC
  R_RT_SCEM : Outport
  LambdaSCEM : Outport  Port=2
  wires:
  LambdaEM/1(Out1) -> LambdaSCEM/1
  R(V)/1 -> R_RT_SCEM/1
  I_ESC_OUT/1 -> Math Function5/1
  T_IN/1 -> Divide3/1
  Aging Velocity1/1 -> Cumulative Aging/1
  Divide3/1 -> Math Function6/1
  Math Function5/1 -> Aging Velocity1/2
  Math Function6/1 -> Aging Velocity1/3
  AeEMSC/1 -> Aging Velocity1/1
  EaEMSC/1 -> Unary Minus2/1
  K/1 -> Divide3/3
  Unary Minus2/1 -> Divide3/2
  NEMSC/1 -> Math Function5/2
  K1/1 -> Divide4/2
  Unary Minus3/1 -> Divide4/1
  TrefEMSC/1 -> Divide4/3
  JrefEMSC/1 -> Math Function7/1
  NEMSC1/1 -> Math Function7/2
  Math Function8/1 -> Veref/3
  Math Function7/1 -> Veref/2
  Divide4/1 -> Math Function8/1
  EaEMSC1/1 -> Unary Minus3/1
  LnomEMSC/1 -> Veref/1
  Cumulative Aging/1 -> Divide2/1, LambdaEM/1(In1)
  Veref/1 -> Divide2/2, LambdaEM/2(In2)
  Unary Minus1/1 -> R(V)/1
  Abs/1 -> Math Function2/1
  Math Function2/1 -> Divide2/3
  Divide2/1 -> Math Function3/1
  Math Function4/1 -> Abs/1
  RrefEMSC/1 -> Math Function4/1
  Unary Minus/1 -> Math Function1/1
  Math Function1/1 -> Math Function2/2
  bEMSC1/1 -> Math Function3/2, Unary Minus/1
  Math Function3/1 -> Unary Minus1/1

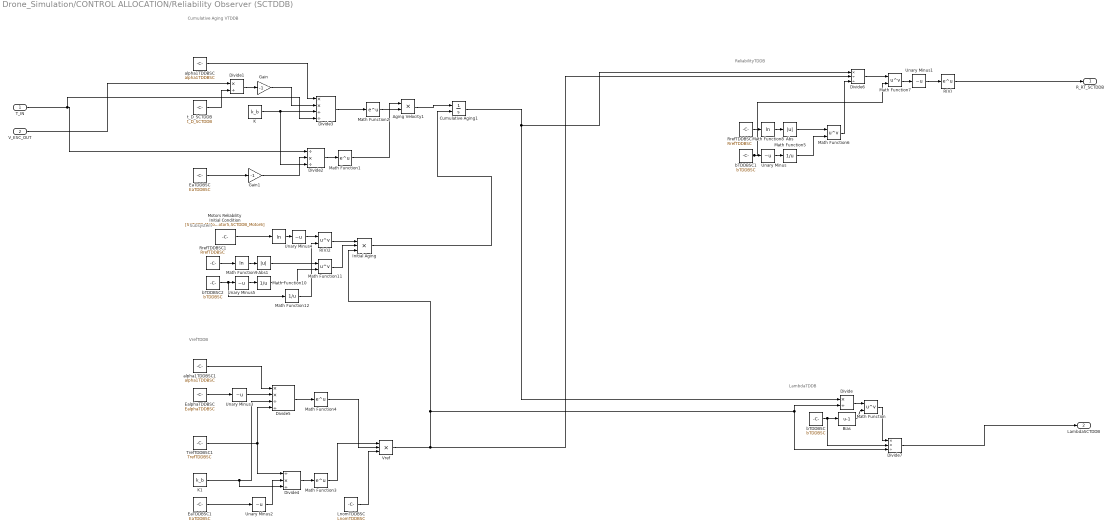
== system Drone_Simulation/CONTROL ALLOCATION/Reliability Observer (SCTDDB) ==
  note: LambdaTDDB
  note: ReliabilityTDDB
  note: VrefTDDB
  note: Cumulative Aging VTDDB
  note: Subsystem
  T_IN : Inport
  V_ESC_OUT : Inport  Port=2
  " " : Math  Operator=log  SaturateOnIntegerOverflow=on
  Abs : Abs
  Abs1 : Abs
  Aging Velocity1 : Product
  Bias : Bias  Bias=-1
  Cumulative Aging1 : Integrator  InitialConditionSource=external
  Divide : Product  Inputs=*/
  Divide1 : Product  Inputs=*/
  Divide2 : Product  Inputs=/*/
  Divide3 : Product  Inputs=**//
  Divide4 : Product  Inputs=/*/
  Divide5 : Product  Inputs=**//
  Divide6 : Product  Inputs=*//
  Divide7 : Product  Inputs=**/
  EaTDDBSC : Constant  Value=EaTDDBSC
  EaTDDBSC1 : Constant  Value=EaTDDBSC
  EalphaTDDBSC : Constant  Value=EalphaTDDBSC
  Gain : Gain  Gain=-1
  Gain1 : Gain  Gain=-1
  Initial Aging : Product  Inputs=3
  K : Constant  Value=k_b  VectorParams1D=off
  K1 : Constant  Value=k_b  VectorParams1D=off
  LnomTDDBSC : Constant  Value=LnomTDDBSC
  Math Function{,6..7,11} (4 alike) : Math  Operator=pow  SaturateOnIntegerOverflow=on
  Math Function{1..4} (4 alike) : Math  SaturateOnIntegerOverflow=on
  Math Function10 : Math  Operator=reciprocal  SaturateOnIntegerOverflow=on
  Math Function12 : Math  Operator=reciprocal  SaturateOnIntegerOverflow=on
  Math Function5 : Math  Operator=reciprocal  SaturateOnIntegerOverflow=on
  Math Function8 : Math  Operator=log  SaturateOnIntegerOverflow=on
  Math Function9 : Math  Operator=log  SaturateOnIntegerOverflow=on
  Motors Reliability Initial Condition : Constant  Value=[SCTDDB_Motor1,SCTDDB_Motor2,SCTDDB_Motor3,SCTDDB_Motor4,SCTDDB_Motor5,SCTDDB_Motor6]
  R(V) : Math  SaturateOnIntegerOverflow=on
  R(V)2 : Math  Operator=pow  SaturateOnIntegerOverflow=on
  RrefTDDBSC : Constant  Value=RrefTDDBSC
  RrefTDDBSC1 : Constant  Value=RrefTDDBSC
  TrefTDDBSC1 : Constant  Value=TrefTDDBSC
  Unary Minus{,1..5} (6 alike) : UnaryMinus
  Vref : Product  Inputs=3
  alpha1TDDBSC : Constant  Value=alpha1TDDBSC
  alpha1TDDBSC1 : Constant  Value=alpha1TDDBSC
  bTDDBSC : Constant  Value=bTDDBSC
  bTDDBSC1 : Constant  Value=bTDDBSC
  bTDDBSC2 : Constant  Value=bTDDBSC
  t_D_SCTDDB : Constant  Value=t_D_SCTDDB
  R_RT_SCTDDB : Outport
  LambdaSCTDDB : Outport  Port=2
  wires:
  R(V)/1 -> R_RT_SCTDDB/1
  Divide7/1 -> LambdaSCTDDB/1
  T_IN/1 -> Divide2/1, Divide3/4
  Aging Velocity1/1 -> Cumulative Aging1/1
  V_ESC_OUT/1 -> Divide1/1
  Divide3/1 -> Math Function2/1
  Divide1/1 -> Gain/1
  t_D_SCTDDB/1 -> Divide1/2
  Divide2/1 -> Math Function1/1
  Math Function2/1 -> Aging Velocity1/2
  EaTDDBSC/1 -> Gain1/1
  K/1 -> Divide3/3, Divide2/3
  Math Function1/1 -> Aging Velocity1/1
  alpha1TDDBSC/1 -> Divide3/1
  Gain/1 -> Divide3/2
  Gain1/1 -> Divide2/2
  Divide4/1 -> Math Function3/1
  Divide5/1 -> Math Function4/1
  Math Function4/1 -> Vref/2
  Math Function3/1 -> Vref/1
  Unary Minus2/1 -> Divide4/2
  EaTDDBSC1/1 -> Unary Minus2/1
  Unary Minus3/1 -> Divide5/2
  LnomTDDBSC/1 -> Vref/3
  TrefTDDBSC1/1 -> Divide5/4, Divide4/1
  alpha1TDDBSC1/1 -> Divide5/1
  EalphaTDDBSC/1 -> Unary Minus3/1
  K1/1 -> Divide4/3, Divide5/3
  Divide6/1 -> Math Function7/1
  Abs/1 -> Math Function6/1
  Math Function7/1 -> Unary Minus1/1
  Math Function6/1 -> Divide6/3
  Math Function8/1 -> Abs/1
  RrefTDDBSC/1 -> Math Function8/1
  Math Function5/1 -> Math Function6/2
  Unary Minus1/1 -> R(V)/1
  bTDDBSC1/1 -> Math Function7/2, Unary Minus/1
  Unary Minus/1 -> Math Function5/1
  Cumulative Aging1/1 -> Divide/1, Divide6/1
  Divide/1 -> Math Function/1
  Math Function/1 -> Divide7/1
  bTDDBSC/1 -> Divide7/2, Bias/1
  Bias/1 -> Math Function/2
  Math Function12/1 -> R(V)2/2
  Math Function10/1 -> Math Function11/2
  R(V)2/1 -> Initial Aging/1
  Math Function9/1 -> Abs1/1
  Abs1/1 -> Math Function11/1
  RrefTDDBSC1/1 -> Math Function9/1
  bTDDBSC2/1 -> Math Function12/1, Unary Minus5/1
  " "/1 -> Unary Minus4/1
  Unary Minus4/1 -> R(V)2/1
  Motors Reliability Initial Condition/1 -> " "/1
  Math Function11/1 -> Initial Aging/2
  Unary Minus5/1 -> Math Function10/1
  Vref/1 -> Divide/2, Divide7/3, Initial Aging/3, Divide6/2
  Initial Aging/1 -> Cumulative Aging1/2

== system Drone_Simulation/CONTROL ALLOCATION/Reliability Observer (SCTDDB)1 ==
  T_IN : Inport
  V_ESC_OUT : Inport  Port=2
  Cumulative Aging VTDDB : Subsystem
  LambdaTDDB : Subsystem
  ReliabilityTDDB : Subsystem
  VrefTDDB : Subsystem
  R_RT_SCTDDB : Outport
  LambdaSCTDDB : Outport  Port=2
  wires:
  V_ESC_OUT/1 -> Cumulative Aging VTDDB/2(V_ESC_OUT)
  LambdaTDDB/1(Out1) -> LambdaSCTDDB/1
  ReliabilityTDDB/1(Out1) -> R_RT_SCTDDB/1
  Cumulative Aging VTDDB/1(Out1) -> LambdaTDDB/1(In1), ReliabilityTDDB/1(In1)
  VrefTDDB/1(Out1) -> LambdaTDDB/2(In2), ReliabilityTDDB/2(In2)
  T_IN/1 -> Cumulative Aging VTDDB/1(T_IN)

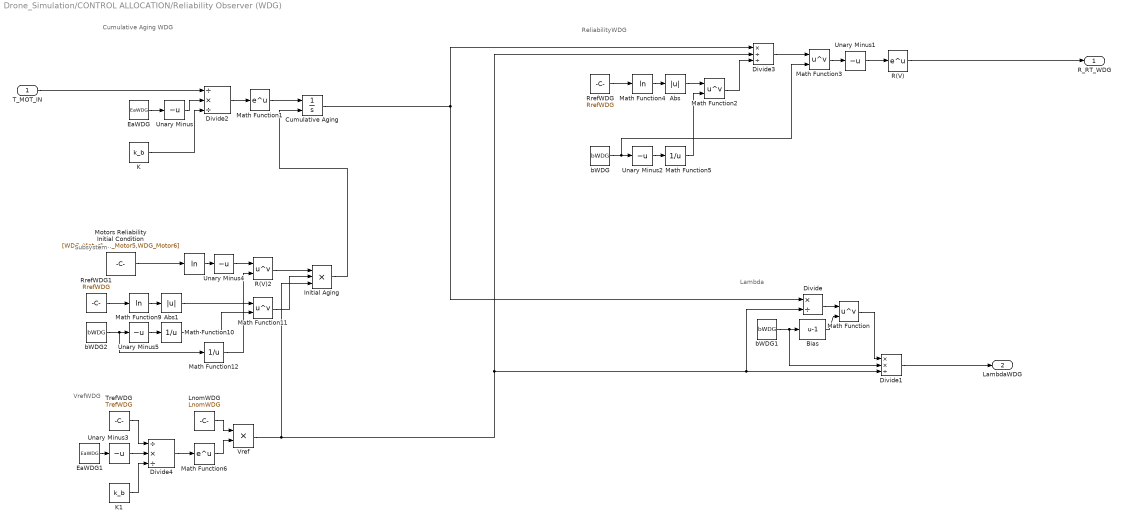
== system Drone_Simulation/CONTROL ALLOCATION/Reliability Observer (WDG) ==
  note: Lambda
  note: ReliabilityWDG
  note: VrefWDG
  note: Cumulative Aging WDG
  note: Subsystem
  T_MOT_IN : Inport
  " " : Math  Operator=log  SaturateOnIntegerOverflow=on
  Abs : Abs
  Abs1 : Abs
  Bias : Bias  Bias=-1
  Cumulative Aging : Integrator  InitialConditionSource=external
  Divide : Product  Inputs=*/
  Divide1 : Product  Inputs=**/
  Divide2 : Product  Inputs=/*/
  Divide3 : Product  Inputs=*//
  Divide4 : Product  Inputs=/*/
  EaWDG : Constant  Value=EaWDG
  EaWDG1 : Constant  Value=EaWDG
  Initial Aging : Product  Inputs=3
  K : Constant  Value=k_b
  K1 : Constant  Value=k_b
  LnomWDG : Constant  Value=LnomWDG
  Math Function{,2..3,11} (4 alike) : Math  Operator=pow  SaturateOnIntegerOverflow=on
  Math Function1 : Math  SaturateOnIntegerOverflow=on
  Math Function10 : Math  Operator=reciprocal  SaturateOnIntegerOverflow=on
  Math Function12 : Math  Operator=reciprocal  SaturateOnIntegerOverflow=on
  Math Function4 : Math  Operator=log  SaturateOnIntegerOverflow=on
  Math Function5 : Math  Operator=reciprocal  SaturateOnIntegerOverflow=on
  Math Function6 : Math  SaturateOnIntegerOverflow=on
  Math Function9 : Math  Operator=log  SaturateOnIntegerOverflow=on
  Motors Reliability Initial Condition : Constant  Value=[WDG_Motor1,WDG_Motor2,WDG_Motor3,WDG_Motor4,WDG_Motor5,WDG_Motor6]
  R(V) : Math  SaturateOnIntegerOverflow=on
  R(V)2 : Math  Operator=pow  SaturateOnIntegerOverflow=on
  RrefWDG : Constant  Value=RrefWDG
  RrefWDG1 : Constant  Value=RrefWDG
  TrefWDG : Constant  Value=TrefWDG
  Unary Minus{,1..5} (6 alike) : UnaryMinus
  Vref : Product
  bWDG : Constant  Value=bWDG
  bWDG1 : Constant  Value=bWDG
  bWDG2 : Constant  Value=bWDG
  R_RT_WDG : Outport
  LambdaWDG : Outport  Port=2
  wires:
  Divide1/1 -> LambdaWDG/1
  R(V)/1 -> R_RT_WDG/1
  T_MOT_IN/1 -> Divide2/1
  Unary Minus/1 -> Divide2/2
  Divide2/1 -> Math Function1/1
  K/1 -> Divide2/3
  EaWDG/1 -> Unary Minus/1
  Math Function1/1 -> Cumulative Aging/1
  TrefWDG/1 -> Divide4/1
  Divide4/1 -> Math Function6/1
  Math Function6/1 -> Vref/2
  LnomWDG/1 -> Vref/1
  K1/1 -> Divide4/3
  Unary Minus3/1 -> Divide4/2
  EaWDG1/1 -> Unary Minus3/1
  Unary Minus2/1 -> Math Function5/1
  Math Function2/1 -> Divide3/3
  RrefWDG/1 -> Math Function4/1
  Math Function5/1 -> Math Function2/2
  Math Function3/1 -> Unary Minus1/1
  bWDG/1 -> Math Function3/2, Unary Minus2/1
  Unary Minus1/1 -> R(V)/1
  Math Function4/1 -> Abs/1
  Abs/1 -> Math Function2/1
  Divide3/1 -> Math Function3/1
  Cumulative Aging/1 -> Divide3/1, Divide/1
  Divide/1 -> Math Function/1
  bWDG1/1 -> Divide1/2, Bias/1
  Math Function/1 -> Divide1/1
  Bias/1 -> Math Function/2
  Vref/1 -> Divide3/2, Divide/2, Divide1/3, Initial Aging/3
  Initial Aging/1 -> Cumulative Aging/2
  Math Function12/1 -> R(V)2/2
  Math Function10/1 -> Math Function11/2
  R(V)2/1 -> Initial Aging/1
  Math Function9/1 -> Abs1/1
  Abs1/1 -> Math Function11/1
  RrefWDG1/1 -> Math Function9/1
  bWDG2/1 -> Math Function12/1, Unary Minus5/1
  " "/1 -> Unary Minus4/1
  Unary Minus4/1 -> R(V)2/1
  Motors Reliability Initial Condition/1 -> " "/1
  Math Function11/1 -> Initial Aging/2
  Unary Minus5/1 -> Math Function10/1

== system Drone_Simulation/CONTROL ALLOCATION/Reliability Observer (WDG)1 ==
  T_MOT_IN : Inport
  Cumulative Aging WDG : Subsystem
  Display : Display
  Lambda : Subsystem
  ReliabilityWDG : Subsystem
  VrefWDG : Subsystem
  R_RT_WDG : Outport
  LambdaWDG : Outport  Port=2
  wires:
  ReliabilityWDG/1(Out1) -> R_RT_WDG/1
  T_MOT_IN/1 -> Cumulative Aging WDG/1(In1)
  Cumulative Aging WDG/1(Out1) -> ReliabilityWDG/1(In1), Lambda/1(In1), Display/1
  VrefWDG/1(Out1) -> ReliabilityWDG/2(In2), Lambda/2(In2)
  Lambda/1(Out1) -> LambdaWDG/1
